simulink model "open_loop"  (R2019b)
settings: Solver=VariableStepAuto  StartTime=0.0  StopTime=10.0  RelTol=1e-3
values from neighbouring files (symbols this model uses):
  A = [[0 1 0]; [a_2/a_1 0 delta]; [-a_2/a_1 0 -M*gamma]]    [controller_tuning.m]
settings Model: Creator=leo  LastModifiedBy=leo

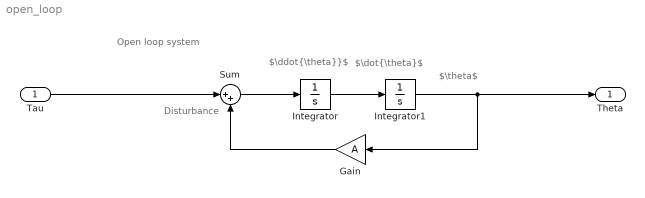
== system open_loop ==
  note: Open loop system
  note: Disturbance
  note: $\ddot{\theta}}$
  note: $\dot{\theta}$
  note: $\theta$
  "Tau " : Inport
  Gain : Gain  Gain=A
  Integrator : Integrator
  Integrator1 : Integrator
  Sum : Sum  Inputs=|++
  Theta : Outport
  wires:
  "Tau "/1 -> Sum/1
  Integrator1/1 -> Gain/1, Theta/1
  Gain/1 -> Sum/2
  Sum/1 -> Integrator/1
  Integrator/1 -> Integrator1/1
